simulink model "BaseEngineController_LS_128"  (Simulink 7.7)
settings: Solver=FixedStepDiscrete  StartTime=0.0  StopTime=10.0  RelTol=1e-3
PreLoadFcn:
  | try, eval([bdroot '_setup']); catch, eval('model_setup', ''); end
InitFcn:
  | try, eval([bdroot '_setup']); catch, eval('model_setup', ''); end
undefined symbols (not defined in the file): ECU565, High, motohawk_build_version, motohawk_trunc_name, motohawk_vardec_config_group, motohawk_vardec_path, True
libraries: MotoHawk_lib x1418, motohawk_control_primitives_lib x183, motohawk_engine_lib x32, simulink x21, motohawk_annotations_lib x9, AutoDoc_lib x8, simulink_extras x4, motohawk_ccp_examples_lib x1, motohawk_control_primitives_motoshare_lib x1
(part 4 of 27)

== system BaseEngineController_LS_128/Main Power Relay/Main Power Relay/On Off Delay ==
  note: Delay the rising and falling of a boolean signal
  In : Inport
  Constant1 : Constant  Value=0  OutDataTypeStr=Inherit: Inherit via back propagation
  Constant2 : Constant  Value=on_delay_count  OutDataTypeStr=Inherit: Inherit via back propagation
  Constant3 : Constant  Value=0  OutDataTypeStr=Inherit: Inherit via back propagation
  Constant4 : Constant  Value=off_delay_count  OutDataTypeStr=Inherit: Inherit via back propagation
  Data Type Conversion : DataTypeConversion  SaturateOnIntegerOverflow=on  RndMeth=Zero
  Data Type Conversion1 : DataTypeConversion  SaturateOnIntegerOverflow=on  RndMeth=Zero
  Logical Operator : Logic  Operator=NOT  AllPortsSameDT=off
  Logical Operator1 : Logic  AllPortsSameDT=off
  Logical Operator2 : Logic  AllPortsSameDT=off
  Relational Operator1 : RelationalOperator
  Relational Operator2 : RelationalOperator
  S-R Flip-Flop : simulink_extras/Flip Flops/S-R Flip-Flop  SystemSampleTime=-1  initial_condition=0
  Sum : Sum  Inputs=|++  SaturateOnIntegerOverflow=on
  Sum1 : Sum  Inputs=|++  SaturateOnIntegerOverflow=on
  Switch : Switch  Threshold=1  SaturateOnIntegerOverflow=on
  Switch1 : Switch  Threshold=1  SaturateOnIntegerOverflow=on
  Terminator : Terminator
  Unit Delay : UnitDelay  SampleTime=-1
  Unit Delay1 : UnitDelay  SampleTime=-1
  Out : Outport
  wires:
  Constant2/1 -> Relational Operator1/2
  Switch/1 -> Relational Operator1/1, Unit Delay/1
  Constant1/1 -> Switch/3
  Sum/1 -> Switch/1
  Data Type Conversion/1 -> Sum/1
  Unit Delay/1 -> Sum/2
  In/1 -> Switch/2, Data Type Conversion/1, Logical Operator2/1, Logical Operator/1
  Switch1/1 -> Unit Delay1/1, Relational Operator2/1
  Constant3/1 -> Switch1/3
  Sum1/1 -> Switch1/1
  Data Type Conversion1/1 -> Sum1/1
  Unit Delay1/1 -> Sum1/2
  Logical Operator/1 -> Data Type Conversion1/1, Switch1/2, Logical Operator1/1
  Constant4/1 -> Relational Operator2/2
  S-R Flip-Flop/1 -> Out/1
  S-R Flip-Flop/2 -> Terminator/1
  Relational Operator2/1 -> Logical Operator1/2
  Relational Operator1/1 -> Logical Operator2/2
  Logical Operator2/1 -> S-R Flip-Flop/1
  Logical Operator1/1 -> S-R Flip-Flop/2

== system BaseEngineController_LS_128/Main Power Relay/Main Power Relay/ShutDown Processes ==
  Manual Reset : Inport
  Input State : Inport  Port=2
  Logical Operator2 : Logic  Operator=OR  AllPortsSameDT=off  OutDataTypeStr=boolean
  Post Shutdown two ticks before MPRD off : Subsystem  TreatAsAtomicUnit=on
  Processor Reboot : Subsystem  TreatAsAtomicUnit=on
  Save NV Vars one tick before MPRD off : Subsystem  TreatAsAtomicUnit=on
  Shutdown power on ECU565/563 : Subsystem  TreatAsAtomicUnit=on
  Unit Delay : UnitDelay  SampleTime=-1
  Unit Delay1 : UnitDelay  SampleTime=-1
  Unit Delay2 : UnitDelay  SampleTime=-1
  motohawk_override_abs : MotoHawk_lib/Calibration & Probing Blocks/motohawk_override_abs  SystemSampleTime=-1  parent_name='MPRD'  parent_val=0  show_more=on  name_source=Use Parameter  parent_read_level=1  parent_override_level=1  view_as=Enumeration  enum_struct={'Off', 'On'}  use_help_units=off  parent_help='Directly Override Main Power Relay'  parent_units='boolean'  use_min_max=off  parent_min=-inf  parent_max=inf  use_precision=off  parent_precision=''  parent_gain=1  parent_offset=0  parent_exp=1  use_mototune_group=on  parent_group=group
  MPRD State : Outport
  wires:
  motohawk_override_abs/1 -> MPRD State/1
  Manual Reset/1 -> Processor Reboot/Enable
  Logical Operator2/1 -> motohawk_override_abs/1
  Unit Delay2/1 -> Logical Operator2/2, Processor Reboot/Trigger
  Input State/1 -> Post Shutdown two ticks before MPRD off/Trigger, Unit Delay/1, Logical Operator2/1
  Unit Delay1/1 -> Unit Delay2/1, Shutdown power on ECU565/563/Trigger
  Unit Delay/1 -> Save NV Vars one tick before MPRD off/Trigger, Unit Delay1/1

== system BaseEngineController_LS_128/Foreground/Control/ActuatorCharacterization/Electronic Throttle Controller ==
  TPS : Inport
  ETCReq : Inport  Port=2
  Enable : EnablePort
  Constant2 : Constant  Value=0  SampleTime=-1
  ETC Adapt Request : Subsystem
  ETC Sticking Fault : Subsystem
  ETC Test  Manager : Stateflow chart  TreatAsAtomicUnit=on
  ETCStallShutDown : Subsystem
  Logical Operator : Logic  Operator=OR  AllPortsSameDT=off  OutDataTypeStr=boolean
  PID With Damper Terms (Tunable) : Subsystem  AncestorBlock=motohawk_control_primitives_lib_new/PID With Damper Terms (Tunable)  mask(PID with Damper Terms (Tunable)){nam='Electronic Throttle Control', prefix='ETC', samp_time=-1, units='%', grp=motohawk_vardec_path(gcb)}
      mask prompts: nam "Name"; samp_time "Sample Time"; grp "MotoTune Group String"
      mask help:
      | This block wraps a 'PID With Damper Terms' block to provide calibrations and probes for most parameters.
      |
      | If 'Sample Time' is -1, then extra code and RAM will be generated to dynamically calculate dt.
      mask Display:
      | patch([0 0 1 1], [0 0.075 0.075 0], [230/255 0/255 0/255])
      | patch([0 0 1 1], [0.025 0.05 0.05 0.025], [150/255 0/255 0/255])
      | patch([0 0 1 1], [0 0.025 0.025 0], [0/255 0/255 0/255])
      | 
      | disp([nam '\n(PIDD)']);
  Relational Operator1 : RelationalOperator  Operator=<  ZeroCross=off  InputSameDT=on
  Relational Operator2 : RelationalOperator  Operator=>  ZeroCross=off  InputSameDT=on
  Relational Operator3 : RelationalOperator  Operator=<  ZeroCross=off  InputSameDT=on
  Relational Operator5 : RelationalOperator  Operator=<  ZeroCross=off  InputSameDT=on
  Reset TasksComplete To True : Subsystem  TreatAsAtomicUnit=on
  Setpoint Manager : Subsystem
  State  Manager : Subsystem
  Switch : Switch  Threshold=1
  Unit Delay : UnitDelay  SampleTime=-1
  motohawk_calibration3 : MotoHawk_lib/Calibration & Probing Blocks/motohawk_calibration  nam='ETC_SpringTestTimerThresh'  val=2  storage=Calibration  show_more=on  name_source=Use Parameter  data_type=double  read_level=1  write_level=1  ovr_cals=on  view_as=Number  enum_struct={'Disabled', 'Enabled'}  vector_style=Wide Row  use_help_units=on  help='During spring test at shutdown, TPS must fall to 0% within this time to prevent fault.'  units='s'  use_header_enum=off  row_header_enum={}  col_header_enum={}  use_min_max=on  min_val=-inf  max_val=inf  use_precision=off  precision=''  gain=1  offset=0  exp=1  use_mototune_group=on  mototune_group=motohawk_vardec_path(gcb)
  motohawk_calibration4 : MotoHawk_lib/Calibration & Probing Blocks/motohawk_calibration  nam='ETC_ShutdownLoAdaptError'  val=-10  storage=Calibration  show_more=on  name_source=Use Parameter  data_type=double  read_level=1  write_level=1  ovr_cals=on  view_as=Number  enum_struct={'Disabled', 'Enabled'}  vector_style=Wide Row  use_help_units=on  help='Drive ETC closed until this error has been achieved in order to catch lo side adapt point.'  units='%'  use_header_enum=off  row_header_enum={}  col_header_enum={}  use_min_max=on  min_val=-inf  max_val=inf  use_precision=off  precision=''  gain=1  offset=0  exp=1  use_mototune_group=on  mototune_group=motohawk_vardec_path(gcb)
  motohawk_calibration5 : MotoHawk_lib/Calibration & Probing Blocks/motohawk_calibration  nam='ETC_SpringTestHiThresh'  val=75  storage=Calibration  show_more=on  name_source=Use Parameter  data_type=double  read_level=1  write_level=1  ovr_cals=on  view_as=Number  enum_struct={'Disabled', 'Enabled'}  vector_style=Wide Row  use_help_units=on  help='Before initiating spring test during shutdown, open the ETC to this setpoint. When achieved, the ETC controller will release the ETC to have the spring close the valve.'  units='%'  use_header_enum=off  row_header_enum={}  col_header_enum={}  use_min_max=on  min_val=-inf  max_val=inf  use_precision=off  precision=''  gain=1  offset=0  exp=1  use_mototune_group=on  mototune_group=motohawk_vardec_path(gcb)
  motohawk_calibration6 : MotoHawk_lib/Calibration & Probing Blocks/motohawk_calibration  nam='ETC_SpringTestLoThresh'  val=40  storage=Calibration  show_more=on  name_source=Use Parameter  data_type=double  read_level=1  write_level=1  ovr_cals=on  view_as=Number  enum_struct={'Disabled', 'Enabled'}  vector_style=Wide Row  use_help_units=on  help='Spring test timer will measure time of travel between ETC_SpringTestHiThresh and ETC_SpringTestLoThresh.'  units='%'  use_header_enum=off  row_header_enum={}  col_header_enum={}  use_min_max=on  min_val=-inf  max_val=inf  use_precision=off  precision=''  gain=1  offset=0  exp=1  use_mototune_group=on  mototune_group=motohawk_vardec_path(gcb)
  motohawk_data_def : MotoHawk_lib/Data Storage Blocks/motohawk_data_def  nam='SpringTestTime'  container_nam=''  data=0  typ=Inherit from 'Initial Value'  struct_nam='MyStruct'  storage=NonVolatile  outputRef=off  use_vardec=off  window=Display  read_level=1  write_level=1  ovr_cals=on  view_as=Number  enum_struct={'Disabled', 'Enabled'}  vector_style=Wide Row  use_help_units=on  help='Time for ETC to close from 80% to 40% at 0% duty cycle.'  units='s'  use_header_enum=off  row_header_enum={}  col_header_enum={}  use_min_max=off  min_val=-inf  max_val=inf  use_precision=off  precision=''  gain=1  offset=0  exp=1  use_mototune_group=on  mototune_group=motohawk_vardec_path(gcb)  eval_name=SpringTestTime  data_stores=motohawk_sfun_data_def_data_stores  struct_instances=motohawk_sfun_data_def_struct_instances  vardecs=motohawk_sfun_data_def_vardecs
  motohawk_data_read : MotoHawk_lib/Data Storage Blocks/motohawk_data_read  source=Lookup By Name  structure=Scalar  operation=Read scalar from location by index  sz_vec=4  sz_row=2  sz_col=3  typ=boolean  nam='ETCStallStateShutdown'  checkNull=on  struct_inst_name='Struct1'  struct_nam='MyStruct'
  motohawk_data_write : MotoHawk_lib/Data Storage Blocks/motohawk_data_write  source=Lookup By Name  structure=Scalar  operation=Write entire data structure at once  sz_vec=-1  sz_row=3  sz_col=2  typ=double  nam='SpringTestTime'  checkNull=off  write_read_only=off  struct_inst_name='Struct1'  struct_name='MyStruct'
  motohawk_fault_def : MotoHawk_lib/Fault Management Blocks/motohawk_fault_def  nam='ETCSpringTest'  mode=Sticky  id=[]  x=1  y=2  input_suspected=on  indeterminate=off  increment_xy=on  downsample_count=1  ovr_cals=on  ovr_actions=on  show_actions=off  action1_name=''  action1_cond=(None)  action2_name=''  action2_cond=(None)  action3_name=''  action3_cond=(None)  action4_name=''  action4_cond=(None)
  ETC : Outport
  ETC_TestActive : Outport  Port=2
  wires:
  motohawk_data_read/1 -> PID With Damper Terms (Tunable)/3(ResetITerm)
  TPS/1 -> Relational Operator2/1, Relational Operator3/1, PID With Damper Terms (Tunable)/1(Actual), Setpoint Manager/1(TPS Position)
  ETCReq/1 -> Setpoint Manager/2(Controller Setpoint)
  ETC Test  Manager/2(DC_Override) -> Logical Operator/1
  Switch/1 -> ETC/1
  State  Manager/2(ECUP Timer) -> ETC Test  Manager/2(Timer)
  ETC Test  Manager/3(TestComplete) -> Reset TasksComplete To True/Trigger
  Relational Operator1/1 -> motohawk_fault_def/1
  Constant2/1 -> Switch/1
  Logical Operator/1 -> ETC_TestActive/1, Switch/2
  PID With Damper Terms (Tunable)/1(Out) -> Switch/3
  Relational Operator2/1 -> ETC Test  Manager/4(TPSHiThresh)
  Relational Operator3/1 -> ETC Test  Manager/5(TPSLoThresh)
  ETC Test  Manager/1(TestTime) -> Relational Operator1/2, motohawk_data_write/1
  motohawk_calibration3/1 -> Relational Operator1/1
  Setpoint Manager/1(ETC_Setpoint) -> PID With Damper Terms (Tunable)/2(SetPoint)
  ETC Test  Manager/4(SetpointMode) -> Setpoint Manager/3(Setpoint Mode), ETC Sticking Fault/2(ETC Setpoint Mode), ETC Adapt Request/1(ETC Setpoint Mode)
  Relational Operator5/1 -> ETC Test  Manager/3(LowAdaptError)
  Unit Delay/1 -> Relational Operator5/1
  State  Manager/1(ECUP State) -> ETC Test  Manager/1(ECUP_Off)
  motohawk_calibration4/1 -> Relational Operator5/2
  motohawk_calibration5/1 -> Relational Operator2/2
  motohawk_calibration6/1 -> Relational Operator3/2
  Setpoint Manager/2(ETC_Error) -> ETC Sticking Fault/1(ETC Error), Unit Delay/1, ETC Adapt Request/2(ETC Error)
  ETCStallShutDown/1(State) -> Logical Operator/2

== system BaseEngineController_LS_128/Foreground/Control/ActuatorCharacterization/Injector Characterization ==
  FPC [mg] : Inport
  BaroPress [kPa] : Inport  Port=2
  MAP [kPa] : Inport  Port=3
  SysVolt09Idx : Inport  Port=4
  RPM : Inport  Port=5
  FuelPress [kPa] : Inport  Port=6
  Constant : Constant  Value=60*1000*2
  DeltaPressureIndex : Subsystem
  Divide : Product  Inputs=*/
  Gain : Gain  Gain=100
  Injector Gain [ms/mg] : MotoHawk_lib/Calibration & Probing Blocks/motohawk_calibration  nam='InjGain'  val=0.351  storage=Calibration  show_more=on  name_source=Use Parameter  data_type=Inherit from 'Default Value'  read_level=1  write_level=1  ovr_cals=on  view_as=Number  enum_struct={'Disabled', 'Enabled'}  vector_style=Wide Row  use_help_units=on  help='Gain value used in the linear transformation of FPC to mechanical pulsewidth.'  units='ms/mg'  use_header_enum=off  row_header_enum={}  col_header_enum={}  use_min_max=off  min_val=0  max_val=inf  use_precision=off  precision='2.4'  gain=1  offset=0  exp=1  use_mototune_group=on  mototune_group=motohawk_vardec_path(gcb)
  Injector Offset [ms] : MotoHawk_lib/Calibration & Probing Blocks/motohawk_calibration  nam='InjOffset'  val=-0.05  storage=Calibration  show_more=on  name_source=Use Parameter  data_type=Inherit from 'Default Value'  read_level=1  write_level=1  ovr_cals=on  view_as=Number  enum_struct={'Disabled', 'Enabled'}  vector_style=Wide Row  use_help_units=on  help='Offset value used in the linear transformation of FPC to mechanical pulsewidth.'  units='ms'  use_header_enum=off  row_header_enum={}  col_header_enum={}  use_min_max=off  min_val=-inf  max_val=inf  use_precision=off  precision='3.4'  gain=1  offset=0  exp=1  use_mototune_group=on  mototune_group=motohawk_vardec_path(gcb)
  MinMax : MinMax  Inputs=2
  Mux1 : Mux  Inputs=3
  Product : Product  Inputs=*/  RndMeth=Zero
  Product2 : Product  SaturateOnIntegerOverflow=on  InputSameDT=on  OutDataTypeStr=Inherit: Same as first input
  Product3 : Product  SaturateOnIntegerOverflow=on  InputSameDT=on  OutDataTypeStr=Inherit: Same as first input
  Saturation : Saturate  UpperLimit=inf  LowerLimit=.01
  Sum : Sum  Inputs=|++  SaturateOnIntegerOverflow=on  InputSameDT=on
  Sum1 : Sum  Inputs=|+-  SaturateOnIntegerOverflow=on
  Sum2 : Sum  Inputs=|-+  SaturateOnIntegerOverflow=on
  motohawk_interpolation_1d1 : MotoHawk_lib/Lookup Tables/motohawk_interpolation_1d  nam='InjTurnOn'  table_data=[1.495 1.293 1.155 1.05 0.968 0.898 0.865 0.823 0.743]  show_more=on  data_type=Inherit from 'Table Data'  storage=NonAdaptive  read_level=1  write_level=1  ovr_cals=on  use_help=on  help='Injector turn on time.'  units='ms'  use_min_max=off  min_val=-inf  max_val=inf  use_precision=off  precision='2.3'  gain=1  offset=0  exp=1  use_links=off  prelookup_block=''  output_name=''  use_mototune_group=on  mototune_group=motohawk_vardec_path(gcb)
  motohawk_interpolation_1d3 : MotoHawk_lib/Lookup Tables/motohawk_interpolation_1d  nam='InjdPComp'  table_data=[1 1 1 1 1 1 1 1 1]  show_more=on  data_type=Inherit from 'Table Data'  storage=NonAdaptive  read_level=1  write_level=1  ovr_cals=on  use_help=on  help='Injector characterization compenastion based on dP across injector.'  units=''  use_min_max=on  min_val=-inf  max_val=inf  use_precision=on  precision='2.3'  gain=1  offset=0  exp=1  use_links=off  prelookup_block=''  output_name=''  use_mototune_group=on  mototune_group=motohawk_vardec_path(gcb)
  motohawk_interpolation_1d4 : MotoHawk_lib/Lookup Tables/motohawk_interpolation_1d  nam='InjTurnOff'  table_data=[0.585 0.583333 0.581667 0.58 0.579167 0.578333 0.576667 0.575833 0.575]  show_more=on  data_type=Inherit from 'Table Data'  storage=NonAdaptive  read_level=1  write_level=1  ovr_cals=on  use_help=on  help='Injector turn off time'  units='ms'  use_min_max=on  min_val=-inf  max_val=inf  use_precision=on  precision='2.3'  gain=1  offset=0  exp=1  use_links=off  prelookup_block=''  output_name=''  use_mototune_group=on  mototune_group=motohawk_vardec_path(gcb)
  motohawk_probe : MotoHawk_lib/Calibration & Probing Blocks/motohawk_probe  nam='InjDC'  show_more=on  name_source=Use Parameter  read_level=1  view_as=Number  enum_struct={'Disabled', 'Enabled'}  vector_style=Wide Row  use_help_units=off  help=''  units=''  use_header_enum=off  row_header_enum={}  col_header_enum={}  use_precision=off  precision=''  gain=1  offset=0  exp=1  use_mototune_group=off  mototune_group=motohawk_vardec_path(gcb)
  motohawk_probe1 : MotoHawk_lib/Calibration & Probing Blocks/motohawk_probe  nam='InjEPW'  show_more=on  name_source=Use Parameter  read_level=1  view_as=Number  enum_struct={'Disabled', 'Enabled'}  vector_style=Wide Row  use_help_units=on  help=''  units=''  use_header_enum=off  row_header_enum={}  col_header_enum={}  use_precision=off  precision=''  gain=1  offset=0  exp=1  use_mototune_group=on  mototune_group=motohawk_vardec_path(gcb)
  motohawk_probe2 : MotoHawk_lib/Calibration & Probing Blocks/motohawk_probe  nam='TotalFPC'  show_more=on  name_source=Use Parameter  read_level=1  view_as=Number  enum_struct={'Disabled', 'Enabled'}  vector_style=Wide Row  use_help_units=on  help='Total fuel per cylinder after application of transient algorithm'  units='mg'  use_header_enum=off  row_header_enum={}  col_header_enum={}  use_precision=off  precision=''  gain=1  offset=0  exp=1  use_mototune_group=on  mototune_group=motohawk_vardec_path(gcb)
  motohawk_probe3 : MotoHawk_lib/Calibration & Probing Blocks/motohawk_probe  nam='InjMPW'  show_more=on  name_source=Use Parameter  read_level=1  view_as=Number  enum_struct={'Disabled', 'Enabled'}  vector_style=Wide Row  use_help_units=on  help=''  units=''  use_header_enum=off  row_header_enum={}  col_header_enum={}  use_precision=off  precision=''  gain=1  offset=0  exp=1  use_mototune_group=on  mototune_group=motohawk_vardec_path(gcb)
  motohawk_probe4 : MotoHawk_lib/Calibration & Probing Blocks/motohawk_probe  nam='MaxAllowableMPW'  show_more=on  name_source=Use Parameter  read_level=1  view_as=Number  enum_struct={'Disabled', 'Enabled'}  vector_style=Wide Row  use_help_units=on  help=''  units=''  use_header_enum=off  row_header_enum={}  col_header_enum={}  use_precision=off  precision=''  gain=1  offset=0  exp=1  use_mototune_group=on  mototune_group=motohawk_vardec_path(gcb)
  MPW [ms] : Outport
  EPWOffset [ms] : Outport  Port=2
  wires:
  DeltaPressureIndex/1(Index) -> motohawk_interpolation_1d3/1, motohawk_interpolation_1d4/1
  Injector Gain [ms/mg]/1 -> Product2/2
  Injector Offset [ms]/1 -> Sum/2
  SysVolt09Idx/1 -> motohawk_interpolation_1d1/1
  motohawk_interpolation_1d1/1 -> Sum2/2
  motohawk_interpolation_1d4/1 -> Sum2/1
  Mux1/1 -> DeltaPressureIndex/1(Inputs)
  BaroPress [kPa]/1 -> Mux1/2
  MAP [kPa]/1 -> Mux1/3
  Sum2/1 -> EPWOffset [ms]/1, Sum1/2, motohawk_probe1/1
  Product2/1 -> Sum/1
  Constant/1 -> Divide/1
  Product3/1 -> MinMax/1
  MinMax/1 -> motohawk_probe3/1, MPW [ms]/1, Product/1
  Sum1/1 -> MinMax/2, motohawk_probe4/1, Product/2
  Divide/1 -> Sum1/1
  RPM/1 -> Saturation/1
  Saturation/1 -> Divide/2
  FuelPress [kPa]/1 -> Mux1/1
  Product/1 -> Gain/1
  Gain/1 -> motohawk_probe/1
  FPC [mg]/1 -> Product2/1, motohawk_probe2/1
  Sum/1 -> Product3/1
  motohawk_interpolation_1d3/1 -> Product3/2

== system BaseEngineController_LS_128/Foreground/Control/ActuatorCharacterization/SequenceCutPattern ==
  Constant : Constant  Value=0  OutDataTypeStr=Inherit: Inherit via back propagation  SampleTime=-1
  Constant1 : Constant  Value=2  OutDataTypeStr=Inherit: Inherit via back propagation  SampleTime=-1
  Constant2 : Constant  OutDataTypeStr=Inherit: Inherit via back propagation  SampleTime=-1
  Constant3 : Constant  Value=2  OutDataTypeStr=Inherit: Inherit via back propagation  SampleTime=-1
  Data Type Conversion2 : DataTypeConversion  SaturateOnIntegerOverflow=on  RndMeth=Zero
  Data Type Conversion3 : DataTypeConversion  SaturateOnIntegerOverflow=on  RndMeth=Zero
  Data Type Conversion4 : DataTypeConversion  SaturateOnIntegerOverflow=on  RndMeth=Zero
  Data Type Conversion5 : DataTypeConversion  OutDataTypeStr=uint8  SaturateOnIntegerOverflow=on  RndMeth=Zero
  Fcn1 : Fcn  Expr=u[1] * 3
  Fcn2 : Fcn  Expr=u[1] * 2
  Fcn3 : Fcn  Expr=u[1] * 1
  Hard Cycle Cut Pattern : Subsystem
  Logical Operator : Logic  Operator=OR
  Logical Operator1 : Logic  Operator=OR
  Logical Operator2 : Logic  Operator=NOT
  Logical Operator3 : Logic  Operator=NOT
  Logical Operator4 : Logic  Operator=OR  Inputs=3  AllPortsSameDT=off
  Medium Cycle Cut Pattern : Subsystem
  Merge1 : Merge  Inputs=3  AllowUnequalInputPortWidths=on
  PassThrough1 : Subsystem  TreatAsAtomicUnit=on
  PassThrough2 : Subsystem  TreatAsAtomicUnit=on
  PassThrough3 : Subsystem  TreatAsAtomicUnit=on
  PassThrough4 : Subsystem  TreatAsAtomicUnit=on
  PassThrough5 : Subsystem  TreatAsAtomicUnit=on
  Relational Operator{,1..3} (4 alike) : RelationalOperator  Operator===  InputSameDT=on
  SequenceCutMachine : Subsystem  TreatAsAtomicUnit=on
      mask Description:
      | When enabled, this block cycles though the 4 input patterns of cylinder disables that can be applied to fuel or spark.
      | 
      | The output should act on the enable inputs for MotoHawk EST and FInj blocks.  Outputs are reset when disabled.
      | 
      | Calibration arrays should be cast as boolean, and can be set up for any cylinder configuration.
      mask Display:
      | patch([0 0 1 1], [0 0.075 0.075 0], [230/255 0/255 0/255])
      | patch([0 0 1 1], [0.025 0.05 0.05 0.025], [150/255 0/255 0/255])
      | patch([0 0 1 1], [0 0.025 0.025 0], [0/255 0/255 0/255])
      | 
      | disp('SEQUENCE DISABLE\nPATTERN');
  Soft Cycle Cut Pattern : Subsystem
  Sum1 : Sum  Inputs=+++  SaturateOnIntegerOverflow=on
  motohawk_calibration1 : MotoHawk_lib/Calibration & Probing Blocks/motohawk_calibration  nam='RevLimitType'  val=0  storage=Calibration  show_more=on  name_source=Use Parameter  data_type=int8  read_level=1  write_level=1  ovr_cals=on  view_as=Enumeration  enum_struct={'Cut Spark', 'Cut Fuel', 'Cut Spark and Fuel'}  vector_style=Wide Row  use_help_units=on  help='Define the type of sequence to be disable when in Rev Limit'  units=''  use_header_enum=off  row_header_enum={}  col_header_enum={}  use_min_max=off  min_val=-inf  max_val=inf  use_precision=off  precision=''  gain=1  offset=0  exp=1  use_mototune_group=on  mototune_group=motohawk_vardec_path(gcb)
  motohawk_fault_action1 : MotoHawk_lib/Fault Management Blocks/motohawk_fault_action  nam='SoftRevLimit'  output_status=on  eval_nam=SoftRevLimit
  motohawk_fault_action2 : MotoHawk_lib/Fault Management Blocks/motohawk_fault_action  nam='MediumRevLimit'  output_status=on  eval_nam=MediumRevLimit
  motohawk_fault_action3 : MotoHawk_lib/Fault Management Blocks/motohawk_fault_action  nam='HardRevLimit'  output_status=on  eval_nam=HardRevLimit
  motohawk_probe42 : MotoHawk_lib/Calibration & Probing Blocks/motohawk_probe  nam='RevLimiterState'  show_more=on  name_source=Use Parameter  read_level=1  view_as=Enumeration  enum_struct={'Disabled', 'Soft', 'Medium', 'Hard'}  vector_style=Wide Row  use_help_units=off  help=''  units=''  use_header_enum=off  row_header_enum={}  col_header_enum={}  use_precision=off  precision=''  gain=1  offset=0  exp=1  use_mototune_group=on  mototune_group=motohawk_vardec_path(gcb)
  Spark : Outport
  Fuel : Outport  Port=2
  wires:
  Logical Operator/1 -> PassThrough4/Enable
  PassThrough4/1(Out1) -> Logical Operator2/1
  PassThrough5/1(Out1) -> Logical Operator3/1
  Logical Operator1/1 -> PassThrough5/Enable
  Relational Operator/1 -> Logical Operator/1
  Relational Operator1/1 -> Logical Operator/2
  motohawk_calibration1/1 -> Relational Operator/1, Relational Operator1/1, Relational Operator2/1, Relational Operator3/1
  Constant/1 -> Relational Operator/2
  Constant1/1 -> Relational Operator1/2
  Constant2/1 -> Relational Operator2/2
  Constant3/1 -> Relational Operator3/2
  Relational Operator2/1 -> Logical Operator1/1
  Relational Operator3/1 -> Logical Operator1/2
  Logical Operator2/1 -> Spark/1
  Logical Operator3/1 -> Fuel/1
  SequenceCutMachine/1(Out1) -> PassThrough4/1(In1), PassThrough5/1(In1)
  Merge1/1 -> SequenceCutMachine/1(Cycles)
  PassThrough1/1(Out1) -> Merge1/1
  motohawk_fault_action1/1 -> PassThrough1/Enable, Logical Operator4/1, Data Type Conversion4/1
  PassThrough2/1(Out1) -> Merge1/2
  motohawk_fault_action2/1 -> PassThrough2/Enable, Logical Operator4/2, Data Type Conversion3/1
  PassThrough3/1(Out1) -> Merge1/3
  motohawk_fault_action3/1 -> PassThrough3/Enable, Logical Operator4/3, Data Type Conversion2/1
  Logical Operator4/1 -> SequenceCutMachine/Enable
  Data Type Conversion2/1 -> Fcn1/1
  Data Type Conversion3/1 -> Fcn2/1
  Data Type Conversion4/1 -> Fcn3/1
  Fcn1/1 -> Sum1/1
  Fcn2/1 -> Sum1/2
  Fcn3/1 -> Sum1/3
  Sum1/1 -> Data Type Conversion5/1
  Data Type Conversion5/1 -> motohawk_probe42/1
  Soft Cycle Cut Pattern/1(Pattern) -> PassThrough1/1(In1)
  Medium Cycle Cut Pattern/1(Pattern) -> PassThrough2/1(In1)
  Hard Cycle Cut Pattern/1(Pattern) -> PassThrough3/1(In1)

== system BaseEngineController_LS_128/Foreground/Control/ActuatorCharacterization/Spark Advance to Start Angle ==
  Stop Angle [degCA] : Inport
  RPM : Inport  Port=2
  PulseWidth [ms] : Inport  Port=3
  Trigger : TriggerPort  TriggerType=function-call
  Product1 : Product  Inputs=**/  SaturateOnIntegerOverflow=on  InputSameDT=on  OutDataTypeStr=Inherit: Same as first input
  Product2 : Product  Inputs=**  SaturateOnIntegerOverflow=on  InputSameDT=on  OutDataTypeStr=Inherit: Same as first input
  Sum : Sum  Inputs=|++  SaturateOnIntegerOverflow=on  InputSameDT=on
  deg/rev : Constant  Value=360
  min/msec : Constant  Value=60000
  Start Angle [degCA] : Outport
  wires:
  Sum/1 -> Start Angle [degCA]/1
  RPM/1 -> Product1/1
  min/msec/1 -> Product1/3
  deg/rev/1 -> Product1/2
  PulseWidth [ms]/1 -> Product2/2  "PulseWidth [ms]"
  Product1/1 -> Product2/1  "deg/ms"
  Product2/1 -> Sum/2  "PulseWidth [degCA]"
  Stop Angle [degCA]/1 -> Sum/1

== system BaseEngineController_LS_128/Foreground/Control/ActuatorCharacterization/Spark Coil Characterization ==
  SparkEnergy [mJ] : Inport
  SysVolt09Idx : Inport  Port=2
  Trigger : TriggerPort  TriggerType=function-call
  Constant : Constant  Value=1000
  Constant1 : Constant  Value=0  OutDataTypeStr=Inherit: Inherit via back propagation
  Only Enable Spark when Energy is Above Zero : RelationalOperator  Operator=>  ZeroCross=off  InputSameDT=on
  Product : Product  Inputs=*/  SaturateOnIntegerOverflow=on  OutDataTypeStr=Inherit: Same as first input
  Sum : Sum  Inputs=|++  SaturateOnIntegerOverflow=on
  motohawk_calibration : MotoHawk_lib/Calibration & Probing Blocks/motohawk_calibration  nam='CoilDrvrDlyTime'  val=0.004  storage=Calibration  show_more=on  name_source=Use Parameter  data_type=Inherit from 'Default Value'  read_level=1  write_level=1  ovr_cals=on  view_as=Number  enum_struct={'Disabled', 'Enabled'}  vector_style=Wide Row  use_help_units=on  help='Coil driver delay time between receipt of EST signal and initiation of coil dwell.'  units='ms'  use_header_enum=off  row_header_enum={}  col_header_enum={}  use_min_max=off  min_val=-inf  max_val=inf  use_precision=off  precision='2.3'  gain=1  offset=0  exp=1  use_mototune_group=on  mototune_group=motohawk_vardec_path(gcb)
  motohawk_interpolation_2d1 : MotoHawk_lib/Lookup Tables/motohawk_interpolation_2d  nam='CoilDwell'  table_data=ones(9)*2  show_more=on  data_type=Inherit from 'Table Data'  storage=NonAdaptive  read_level=1  write_level=1  ovr_cals=on  use_help=on  help='Required spark dwell to give the desired spark energy.'  units='ms'  use_min_max=on  min_val=-inf  max_val=inf  use_precision=on  precision=''  gain=1  offset=0  exp=1  use_links=off  row_prelookup_block=''  col_prelookup_block=''  output_name=''  use_mototune_group=on  mototune_group=motohawk_vardec_path(gcb)
  motohawk_override_rel : MotoHawk_lib/Calibration & Probing Blocks/motohawk_override_rel  SystemSampleTime=-1  parent_name='SparkDwell'  show_more=on  name_source=Use Parameter  parent_read_level=1  parent_override_level=1  use_help_units=off  parent_help=''  parent_units=''  use_min_max=off  parent_min=-inf  parent_max=inf  use_precision=off  parent_precision=''  parent_gain=1  parent_offset=0  parent_exp=1  use_mototune_group=on  parent_group=motohawk_vardec_path(gcb)
  motohawk_prelookup : MotoHawk_lib/Lookup Tables/motohawk_prelookup  nam='SpkEnergy09'  breakpoint_data=[10 19 29 38 48 57 66 76 86]  show_more=on  data_type=Inherit from 'Table Data'  storage=Constant  read_level=1  write_level=1  ovr_cals=on  use_help=on  help=''  units=''  use_min_max=off  min_val=-inf  max_val=inf  use_precision=on  precision=''  gain=1  offset=0  exp=1  use_links=off  input_name=''  use_mototune_group=on  mototune_group=motohawk_vardec_path(gcb)
  motohawk_probe : MotoHawk_lib/Calibration & Probing Blocks/motohawk_probe  nam='SparkDwell'  show_more=on  name_source=Use Parameter  read_level=1  view_as=Number  enum_struct={'Disabled', 'Enabled'}  vector_style=Wide Row  use_help_units=on  help='Total electrical spark dwell time'  units='ms'  use_header_enum=off  row_header_enum={}  col_header_enum={}  use_precision=off  precision=''  gain=1  offset=0  exp=1  use_mototune_group=on  mototune_group=motohawk_vardec_path(gcb)
  motohawk_probe1 : MotoHawk_lib/Calibration & Probing Blocks/motohawk_probe  nam='SparkEnergyMonitor'  show_more=on  name_source=Use Parameter  read_level=1  view_as=Number  enum_struct={'Disabled', 'Enabled'}  vector_style=Wide Row  use_help_units=on  help='Commanded spark energy, before conversion to dwell time'  units='mJ'  use_header_enum=off  row_header_enum={}  col_header_enum={}  use_precision=off  precision=''  gain=1  offset=0  exp=1  use_mototune_group=on  mototune_group=motohawk_vardec_path(gcb)
  motohawk_probe2 : MotoHawk_lib/Calibration & Probing Blocks/motohawk_probe  nam='SparkEnabled'  show_more=on  name_source=Use Parameter  read_level=1  view_as=Number  enum_struct={'Disabled', 'Enabled'}  vector_style=Wide Row  use_help_units=on  help='Enabled when spark energy is greater than zero'  units='boolean'  use_header_enum=off  row_header_enum={}  col_header_enum={}  use_precision=off  precision=''  gain=1  offset=0  exp=1  use_mototune_group=on  mototune_group=motohawk_vardec_path(gcb)
  SparkDwell [ms] : Outport
  SparkEnable [bool] : Outport  Port=2
  wires:
  SysVolt09Idx/1 -> motohawk_interpolation_2d1/2  "SysVolt10Idx"
  motohawk_prelookup/1 -> motohawk_interpolation_2d1/1  "SpkEnergy09Idx"
  SparkEnergy [mJ]/1 -> motohawk_probe1/1, Only Enable Spark when Energy is Above Zero/1, motohawk_prelookup/1
  Sum/1 -> motohawk_override_rel/1
  motohawk_calibration/1 -> Product/1
  Product/1 -> Sum/2
  Constant/1 -> Product/2
  Only Enable Spark when Energy is Above Zero/1 -> SparkEnable [bool]/1, motohawk_probe2/1
  Constant1/1 -> Only Enable Spark when Energy is Above Zero/2
  motohawk_override_rel/1 -> motohawk_probe/1, SparkDwell [ms]/1
  motohawk_interpolation_2d1/1 -> Sum/1

== system BaseEngineController_LS_128/Foreground/Control/Controller/Crank ==
  Inputs : Inport
  Enable : EnablePort  StatesWhenEnabling=reset
  Bus Creator2 : BusCreator  Inputs=13
  Bus Selector : BusSelector  OutputSignals=Raw.RPM,Raw.NonLinearSensors.ECT,RawProcessed.APP1,RawProcessed.TPS,Raw.NonLinearSensors.IAT,Raw.LinearSensors.FuelSense
  CrankFueling : Subsystem
  CrankIAC : Subsystem
  Data Type Conversion : DataTypeConversion  OutDataTypeStr=double
  Data Type Conversion1 : DataTypeConversion  OutDataTypeStr=double
  Data Type Conversion2 : DataTypeConversion  OutDataTypeStr=double
  IAC Characterization : Subsystem
  Mult1 : Constant  Value=0  OutDataTypeStr=double
  Mult2 : Constant  Value=0  OutDataTypeStr=double
  OFF : Constant  Value=0  OutDataTypeStr=boolean
  OFF3 : Constant  Value=0  OutDataTypeStr=boolean
  ON : Constant  OutDataTypeStr=boolean
  Zero-Order Hold{1..9,11..14} (13 alike) : ZeroOrderHold  SampleTime=-1
  motohawk_interpolation_1d1 : MotoHawk_lib/Lookup Tables/motohawk_interpolation_1d  nam='CrankAirflowSetPt'  table_data=[34 34 34 31 30]  show_more=on  data_type=Inherit from 'Table Data'  storage=NonAdaptive  read_level=1  write_level=1  ovr_cals=on  use_help=on  help='ETC setpoint during cranking.'  units='%'  use_min_max=off  min_val=-inf  max_val=inf  use_precision=off  precision=''  gain=1  offset=0  exp=1  use_links=off  prelookup_block=''  output_name=''  use_mototune_group=on  mototune_group=motohawk_vardec_path(gcb)
  motohawk_interpolation_1d4 : MotoHawk_lib/Lookup Tables/motohawk_interpolation_1d  nam='CrankSOI'  table_data=[500 500 500 500 500]  show_more=on  data_type=Inherit from 'Table Data'  storage=NonAdaptive  read_level=1  write_level=1  ovr_cals=on  use_help=on  help='Start of injection during cranking.'  units='degBTDC'  use_min_max=on  min_val=-920  max_val=920  use_precision=on  precision=''  gain=1  offset=0  exp=1  use_links=off  prelookup_block=''  output_name=''  use_mototune_group=on  mototune_group=motohawk_vardec_path(gcb)
  motohawk_interpolation_1d5 : MotoHawk_lib/Lookup Tables/motohawk_interpolation_1d  nam='CrankMakeUpEOI'  table_data=[200 200 200 200 200]  show_more=on  data_type=Inherit from 'Table Data'  storage=NonAdaptive  read_level=1  write_level=1  ovr_cals=on  use_help=on  help='Start of injection during cranking.'  units='degBTDC'  use_min_max=on  min_val=-920  max_val=920  use_precision=on  precision=''  gain=1  offset=0  exp=1  use_links=off  prelookup_block=''  output_name=''  use_mototune_group=on  mototune_group=motohawk_vardec_path(gcb)
  motohawk_interpolation_2d : MotoHawk_lib/Lookup Tables/motohawk_interpolation_2d  nam='CrankSpark'  table_data=ones(5,5)  show_more=on  data_type=Inherit from 'Table Data'  storage=NonAdaptive  read_level=1  write_level=1  ovr_cals=on  use_help=on  help='Spark adv during cranking.'  units='degBTDC'  use_min_max=on  min_val=-100  max_val=100  use_precision=off  precision=''  gain=1  offset=0  exp=1  use_links=off  row_prelookup_block=''  col_prelookup_block=''  output_name=''  use_mototune_group=on  mototune_group=motohawk_vardec_path(gcb)
  motohawk_interpolation_2d1 : MotoHawk_lib/Lookup Tables/motohawk_interpolation_2d  nam='CrankSpkEnergy'  table_data=[80 72.5 65 57 50;80 72.5 65 57.5 50;80 72.5 65 57.5 50;80 72.5 65 57.5 50;80 72.5 65 57.5 50]  show_more=on  data_type=Inherit from 'Table Data'  storage=NonAdaptive  read_level=1  write_level=1  ovr_cals=on  use_help=on  help='Spark energy during cranking.'  units='MJ'  use_min_max=on  min_val=0  max_val=inf  use_precision=on  precision=''  gain=1  offset=0  exp=1  use_links=off  row_prelookup_block=''  col_prelookup_block=''  output_name=''  use_mototune_group=on  mototune_group=motohawk_vardec_path(gcb)
  motohawk_prelookup : MotoHawk_lib/Lookup Tables/motohawk_prelookup  nam='CrankRPM05'  breakpoint_data=[0 100 200 400 500]  show_more=on  data_type=Inherit from 'Table Data'  storage=Constant  read_level=1  write_level=1  ovr_cals=on  use_help=on  help='RPM pre-lookup for crank maps'  units='RPM'  use_min_max=off  min_val=-inf  max_val=inf  use_precision=off  precision=''  gain=1  offset=0  exp=1  use_links=on  input_name=''  use_mototune_group=on  mototune_group=motohawk_vardec_path(gcb)
  motohawk_prelookup1 : MotoHawk_lib/Lookup Tables/motohawk_prelookup  nam='CrankECT05'  breakpoint_data=[-40 -3.75 32.5 68.75 105]  show_more=on  data_type=Inherit from 'Table Data'  storage=Constant  read_level=1  write_level=1  ovr_cals=on  use_help=on  help='ECT pre-lookup for crank maps.'  units='degC'  use_min_max=off  min_val=-inf  max_val=inf  use_precision=off  precision=''  gain=1  offset=0  exp=1  use_links=on  input_name='ECT'  use_mototune_group=on  mototune_group=motohawk_vardec_path(gcb)
  motohawk_prelookup2 : MotoHawk_lib/Lookup Tables/motohawk_prelookup  nam='CrankIAT05'  breakpoint_data=[-40 -3.75 32.5 68.75 105]  show_more=on  data_type=Inherit from 'Table Data'  storage=Constant  read_level=1  write_level=1  ovr_cals=on  use_help=on  help='IAT pre-lookup for crank maps.'  units='degC'  use_min_max=off  min_val=-inf  max_val=inf  use_precision=off  precision=''  gain=1  offset=0  exp=1  use_links=on  input_name='IAT'  use_mototune_group=on  mototune_group=motohawk_vardec_path(gcb)
  motohawk_prelookup3 : MotoHawk_lib/Lookup Tables/motohawk_prelookup  nam='CrankOXY05'  breakpoint_data=[0 25 50 75 100]  show_more=on  data_type=Inherit from 'Table Data'  storage=Constant  read_level=1  write_level=1  ovr_cals=on  use_help=on  help='OXY pre-lookup for crank maps.'  units='%'  use_min_max=off  min_val=-inf  max_val=inf  use_precision=off  precision=''  gain=1  offset=0  exp=1  use_links=off  input_name=''  use_mototune_group=on  mototune_group=motohawk_vardec_path(gcb)
  motohawk_replicate : MotoHawk_lib/Extra Development Blocks/motohawk_replicate  output_width=-1
  motohawk_replicate1 : MotoHawk_lib/Extra Development Blocks/motohawk_replicate  output_width=-1
  Actuators : Outport
  wires:
  Inputs/1 -> Bus Selector/1
  motohawk_prelookup1/1 -> CrankFueling/2(ECTIdx), motohawk_interpolation_2d1/1, motohawk_interpolation_2d/1, motohawk_interpolation_1d1/1, CrankIAC/2(ECTIdx)
  motohawk_prelookup/1 -> motohawk_interpolation_1d4/1, motohawk_interpolation_1d5/1, motohawk_interpolation_2d1/2, motohawk_interpolation_2d/2, CrankIAC/1(RPMIdx), CrankFueling/1(RPMIdx)
  Bus Selector/2 -> motohawk_prelookup1/1  "<ECT>"
  Bus Selector/1 -> motohawk_prelookup/1  "<RPM>"
  CrankFueling/1(FPC) -> motohawk_replicate/1
  Zero-Order Hold6/1 -> Bus Creator2/1  "FPC"
  Zero-Order Hold5/1 -> Bus Creator2/2  "SOI"
  ON/1 -> Zero-Order Hold7/1
  motohawk_interpolation_1d1/1 -> Zero-Order Hold9/1
  motohawk_interpolation_1d4/1 -> Zero-Order Hold5/1
  Zero-Order Hold4/1 -> Bus Creator2/4  "SparkEnergy"
  Zero-Order Hold3/1 -> Bus Creator2/5  "SparkAdv"
  Zero-Order Hold9/1 -> Bus Creator2/6  "Throttle"
  Zero-Order Hold7/1 -> Bus Creator2/7  "FUELP"
  motohawk_replicate/1 -> Zero-Order Hold6/1
  motohawk_interpolation_1d5/1 -> Zero-Order Hold8/1
  Zero-Order Hold8/1 -> Bus Creator2/3  "EOI"
  motohawk_replicate1/1 -> Zero-Order Hold3/1
  Bus Selector/3 -> CrankFueling/3(APP)  "<APP1>"
  motohawk_interpolation_2d1/1 -> Zero-Order Hold4/1
  Bus Selector/4 -> CrankFueling/4(TPS)  "<TPS>"
  Bus Creator2/1 -> Actuators/1
  Zero-Order Hold1/1 -> Data Type Conversion/1  "IAC-P"
  Zero-Order Hold2/1 -> Data Type Conversion1/1  "IAC-S"
  OFF/1 -> Zero-Order Hold11/1
  Zero-Order Hold11/1 -> Data Type Conversion2/1  "WASTEGATE"
  Bus Selector/5 -> motohawk_prelookup2/1  "<IAT>"
  motohawk_prelookup2/1 -> CrankFueling/5(IATIdx), CrankIAC/3(IATIdx)
  Bus Selector/6 -> motohawk_prelookup3/1  "<FuelSense>"
  motohawk_prelookup3/1 -> CrankFueling/6(OXYIdx), CrankIAC/4(OXYIdx)
  motohawk_interpolation_2d/1 -> motohawk_replicate1/1
  CrankIAC/1(IAC %) -> IAC Characterization/1(IAC %)
  IAC Characterization/2(IAC-S) -> Zero-Order Hold2/1
  IAC Characterization/1(IAC-P) -> Zero-Order Hold1/1
  Mult1/1 -> Zero-Order Hold12/1
  Mult2/1 -> Zero-Order Hold13/1
  OFF3/1 -> Zero-Order Hold14/1
  Data Type Conversion/1 -> Bus Creator2/8  "IAC-P"
  Data Type Conversion1/1 -> Bus Creator2/9  "IAC-S"
  Data Type Conversion2/1 -> Bus Creator2/10  "WASTEGATE"
  Zero-Order Hold12/1 -> Bus Creator2/11  "FAN-1"
  Zero-Order Hold13/1 -> Bus Creator2/12  "FAN-2"
  Zero-Order Hold14/1 -> Bus Creator2/13  "AC"

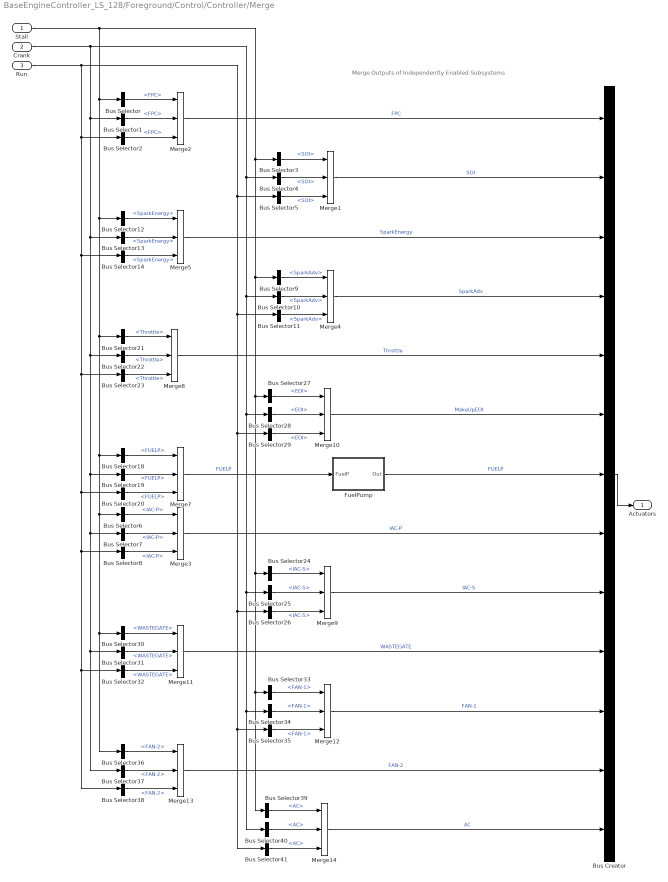
== system BaseEngineController_LS_128/Foreground/Control/Controller/Merge ==
  note: Merge Outputs of Independently Enabled Subsystems
  Stall : Inport
  Crank : Inport  Port=2
  Run : Inport  Port=3
  Bus Creator : BusCreator  Inputs=13
  Bus Selector : BusSelector  OutputSignals=FPC
  Bus Selector1 : BusSelector  OutputSignals=FPC
  Bus Selector10 : BusSelector  OutputSignals=SparkAdv
  Bus Selector11 : BusSelector  OutputSignals=SparkAdv
  Bus Selector12 : BusSelector  OutputSignals=SparkEnergy
  Bus Selector13 : BusSelector  OutputSignals=SparkEnergy
  Bus Selector14 : BusSelector  OutputSignals=SparkEnergy
  Bus Selector18 : BusSelector  OutputSignals=FUELP
  Bus Selector19 : BusSelector  OutputSignals=FUELP
  Bus Selector2 : BusSelector  OutputSignals=FPC
  Bus Selector20 : BusSelector  OutputSignals=FUELP
  Bus Selector21 : BusSelector  OutputSignals=Throttle
  Bus Selector22 : BusSelector  OutputSignals=Throttle
  Bus Selector23 : BusSelector  OutputSignals=Throttle
  Bus Selector24 : BusSelector  OutputSignals=IAC-S
  Bus Selector25 : BusSelector  OutputSignals=IAC-S
  Bus Selector26 : BusSelector  OutputSignals=IAC-S
  Bus Selector27 : BusSelector  OutputSignals=EOI
  Bus Selector28 : BusSelector  OutputSignals=EOI
  Bus Selector29 : BusSelector  OutputSignals=EOI
  Bus Selector3 : BusSelector  OutputSignals=SOI
  Bus Selector30 : BusSelector  OutputSignals=WASTEGATE
  Bus Selector31 : BusSelector  OutputSignals=WASTEGATE
  Bus Selector32 : BusSelector  OutputSignals=WASTEGATE
  Bus Selector33 : BusSelector  OutputSignals=FAN-1
  Bus Selector34 : BusSelector  OutputSignals=FAN-1
  Bus Selector35 : BusSelector  OutputSignals=FAN-1
  Bus Selector36 : BusSelector  OutputSignals=FAN-2
  Bus Selector37 : BusSelector  OutputSignals=FAN-2
  Bus Selector38 : BusSelector  OutputSignals=FAN-2
  Bus Selector39 : BusSelector  OutputSignals=AC
  Bus Selector4 : BusSelector  OutputSignals=SOI
  Bus Selector40 : BusSelector  OutputSignals=AC
  Bus Selector41 : BusSelector  OutputSignals=AC
  Bus Selector5 : BusSelector  OutputSignals=SOI
  Bus Selector6 : BusSelector  OutputSignals=IAC-P
  Bus Selector7 : BusSelector  OutputSignals=IAC-P
  Bus Selector8 : BusSelector  OutputSignals=IAC-P
  Bus Selector9 : BusSelector  OutputSignals=SparkAdv
  FuelPump : Subsystem
  Merge{1..5,7..14} (13 alike) : Merge  Inputs=3
  Actuators : Outport
  wires:
  Bus Selector23/1 -> Merge8/3  "<Throttle>"
  Bus Selector22/1 -> Merge8/2  "<Throttle>"
  Bus Selector21/1 -> Merge8/1  "<Throttle>"
  Bus Selector20/1 -> Merge7/3  "<FUELP>"
  Bus Selector19/1 -> Merge7/2  "<FUELP>"
  Bus Selector18/1 -> Merge7/1  "<FUELP>"
  Merge7/1 -> FuelPump/1(FuelP)  "FUELP"
  Bus Selector14/1 -> Merge5/3  "<SparkEnergy>"
  Bus Selector13/1 -> Merge5/2  "<SparkEnergy>"
  Bus Selector12/1 -> Merge5/1  "<SparkEnergy>"
  Bus Selector11/1 -> Merge4/3  "<SparkAdv>"
  Bus Selector10/1 -> Merge4/2  "<SparkAdv>"
  Bus Selector9/1 -> Merge4/1  "<SparkAdv>"
  Bus Selector5/1 -> Merge1/3  "<SOI>"
  Bus Selector4/1 -> Merge1/2  "<SOI>"
  Bus Selector3/1 -> Merge1/1  "<SOI>"
  Run/1 -> Bus Selector11/1, Bus Selector29/1, Bus Selector26/1, Bus Selector35/1, Bus Selector41/1, Bus Selector5/1, Bus Selector2/1, Bus Selector14/1, Bus Selector23/1, Bus Selector20/1, Bus Selector8/1, Bus Selector32/1, Bus Selector38/1
  Crank/1 -> Bus Selector10/1, Bus Selector28/1, Bus Selector25/1, Bus Selector34/1, Bus Selector40/1, Bus Selector4/1, Bus Selector1/1, Bus Selector13/1, Bus Selector22/1, Bus Selector19/1, Bus Selector7/1, Bus Selector31/1, Bus Selector37/1
  Stall/1 -> Bus Selector9/1, Bus Selector27/1, Bus Selector24/1, Bus Selector33/1, Bus Selector39/1, Bus Selector3/1, Bus Selector/1, Bus Selector12/1, Bus Selector21/1, Bus Selector18/1, Bus Selector6/1, Bus Selector30/1, Bus Selector36/1
  Bus Creator/1 -> Actuators/1
  Bus Selector/1 -> Merge2/1  "<FPC>"
  Bus Selector1/1 -> Merge2/2  "<FPC>"
  Bus Selector2/1 -> Merge2/3  "<FPC>"
  Merge2/1 -> Bus Creator/1  "FPC"
  Merge1/1 -> Bus Creator/2  "SOI"
  Merge5/1 -> Bus Creator/3  "SparkEnergy"
  Merge8/1 -> Bus Creator/5  "Throttle"
  Merge4/1 -> Bus Creator/4  "SparkAdv"
  FuelPump/1(Out) -> Bus Creator/7  "FUELP"
  Bus Selector29/1 -> Merge10/3  "<EOI>"
  Bus Selector28/1 -> Merge10/2  "<EOI>"
  Bus Selector27/1 -> Merge10/1  "<EOI>"
  Merge10/1 -> Bus Creator/6  "MakeUpEOI"
  Bus Selector8/1 -> Merge3/3  "<IAC-P>"
  Bus Selector7/1 -> Merge3/2  "<IAC-P>"
  Bus Selector6/1 -> Merge3/1  "<IAC-P>"
  Bus Selector26/1 -> Merge9/3  "<IAC-S>"
  Bus Selector25/1 -> Merge9/2  "<IAC-S>"
  Bus Selector24/1 -> Merge9/1  "<IAC-S>"
  Bus Selector32/1 -> Merge11/3  "<WASTEGATE>"
  Bus Selector31/1 -> Merge11/2  "<WASTEGATE>"
  Bus Selector30/1 -> Merge11/1  "<WASTEGATE>"
  Bus Selector35/1 -> Merge12/3  "<FAN-1>"
  Bus Selector34/1 -> Merge12/2  "<FAN-1>"
  Bus Selector33/1 -> Merge12/1  "<FAN-1>"
  Bus Selector38/1 -> Merge13/3  "<FAN-2>"
  Bus Selector37/1 -> Merge13/2  "<FAN-2>"
  Bus Selector36/1 -> Merge13/1  "<FAN-2>"
  Bus Selector41/1 -> Merge14/3  "<AC>"
  Bus Selector40/1 -> Merge14/2  "<AC>"
  Bus Selector39/1 -> Merge14/1  "<AC>"
  Merge3/1 -> Bus Creator/8  "IAC-P"
  Merge9/1 -> Bus Creator/9  "IAC-S"
  Merge11/1 -> Bus Creator/10  "WASTEGATE"
  Merge12/1 -> Bus Creator/11  "FAN-1"
  Merge13/1 -> Bus Creator/12  "FAN-2"
  Merge14/1 -> Bus Creator/13  "AC"

== system BaseEngineController_LS_128/Foreground/Control/Controller/Run ==
  Inputs : Inport
  Enable : EnablePort  StatesWhenEnabling=reset  ShowOutputPort=on
  AC Control : Subsystem
  AirFlow Manager : Subsystem
  Base Equiv Ratio : Subsystem  TreatAsAtomicUnit=on
  Boost Control : Subsystem
  Bus Creator2 : BusCreator  Inputs=13
  DFCO : Subsystem
  Demux : Demux  Outputs=7
  FAN Control : Subsystem
  Fuel System Manager : Subsystem  TreatAsAtomicUnit=on
  IAC Characterization : Subsystem
  MaxGovernor : Subsystem  TreatAsAtomicUnit=on
  MinGovernor : Subsystem  TreatAsAtomicUnit=on
  O2 Control : Subsystem  TreatAsAtomicUnit=on
  ON1 : Constant  OutDataTypeStr=boolean
  Spark Manager : Subsystem  TreatAsAtomicUnit=on
  Zero-Order Hold{1..3,5..9,11..12,16..18} (13 alike) : ZeroOrderHold  SampleTime=-1
  motohawk_trigger1 : MotoHawk_lib/Trigger Blocks/motohawk_trigger  Tag=Trigger  trigger=FGND_5XRTI_PERIODIC  function_name=Trigger_FGND_5XRTI_PERIODIC_5057p0001  priority_order=1  inherited=on  run_disabled=off  override_app_monitor=off  target=ECU565_128
  Actuators : Outport
  DesEquivRatio : Outport  Port=2
  wires:
  Enable/1 -> O2 Control/1(Reset)
  Inputs/1 -> Base Equiv Ratio/1(Sensors), Spark Manager/2(Sensors), MinGovernor/1(Sensors), MaxGovernor/2(Sensors), AirFlow Manager/3(Sensors), Boost Control/1(Sensors), FAN Control/1(Sensors), AC Control/1(Sensors), DFCO/2(Sensors), O2 Control/2(Sensors), Fuel System Manager/1(Sensors)
  ON1/1 -> Zero-Order Hold16/1  "FUELP"
  Bus Creator2/1 -> Actuators/1
  Spark Manager/1(SparkEnergy) -> Zero-Order Hold1/1  "SparkEnergy"
  MinGovernor/1(MinGovInfo) -> Spark Manager/3(RPM_Ctrl_Ofst), AirFlow Manager/1(MinGovInfo), IAC Characterization/1(MinGovINFO), MaxGovernor/1(MinGovInfo)
  Spark Manager/2(SpkAdv) -> Zero-Order Hold12/1  "SparkAdv"
  MaxGovernor/1(MaxGovInfo) -> AirFlow Manager/2(MaxGovInfo)
  Fuel System Manager/1(DesiredFuel) -> Zero-Order Hold9/1  "FPC"
  Fuel System Manager/2(InjTiming) -> Zero-Order Hold17/1  "SOI"
  Fuel System Manager/3(EOI) -> Zero-Order Hold3/1  "EOI"
  O2 Control/1(O2_Info) -> Fuel System Manager/2(O2_Info)
  Zero-Order Hold3/1 -> Bus Creator2/3  "EOI"
  Zero-Order Hold17/1 -> Bus Creator2/2  "SOI"
  motohawk_trigger1/1 -> Demux/1
  IAC Characterization/2(IAC-S) -> Zero-Order Hold5/1
  IAC Characterization/1(IAC-P) -> Zero-Order Hold2/1
  Boost Control/1(Wastegate) -> Zero-Order Hold11/1
  FAN Control/1(FAN-1) -> Zero-Order Hold6/1
  FAN Control/2(FAN-2) -> Zero-Order Hold7/1
  AC Control/1(AC) -> Zero-Order Hold8/1, MinGovernor/2(AC)
  AirFlow Manager/1(ETC%) -> Zero-Order Hold18/1  "Throttle"
  Base Equiv Ratio/1(EquivRatioInfo) -> DFCO/1(EquivRatioInfo)
  DFCO/1(DesEquivRatio) -> O2 Control/3(Desired_Equiv), Spark Manager/1(DesEquivRatio), DesEquivRatio/1
  DFCO/2(DFCOInfo) -> Spark Manager/4(DFCOInfo)
  Demux/1 -> DFCO/Trigger
  Demux/2 -> MinGovernor/Trigger
  Demux/3 -> AC Control/Trigger
  Demux/4 -> Boost Control/Trigger
  Demux/5 -> FAN Control/Trigger
  Demux/6 -> MaxGovernor/Trigger
  Demux/7 -> Spark Manager/Trigger
  Zero-Order Hold9/1 -> Bus Creator2/1  "FPC"
  Zero-Order Hold1/1 -> Bus Creator2/4  "SparkEnergy"
  Zero-Order Hold12/1 -> Bus Creator2/5  "SparkAdv"
  Zero-Order Hold18/1 -> Bus Creator2/6  "Throttle"
  Zero-Order Hold16/1 -> Bus Creator2/7  "FUELP"
  Zero-Order Hold2/1 -> Bus Creator2/8  "IAC-P"
  Zero-Order Hold5/1 -> Bus Creator2/9  "IAC-S"
  Zero-Order Hold11/1 -> Bus Creator2/10  "WASTEGATE"
  Zero-Order Hold6/1 -> Bus Creator2/11  "FAN-1"
  Zero-Order Hold7/1 -> Bus Creator2/12  "FAN-2"
  Zero-Order Hold8/1 -> Bus Creator2/13  "AC"
